simulink model "decibel"  (R2018a)
settings: Solver=VariableStepAuto  StartTime=0.0  StopTime=10e-3  RelTol=1e-3
libraries: simulink x1
settings Model: Creator=alex8  LastModifiedBy=alex8
settings OptimizationCC: DefaultParameterBehavior=Inlined  UseDivisionForNetSlopeComputation=on  UseFloatMulNetSlope=on  UseSpecifiedMinMax=on  InlineInvariantSignals=on  PassReuseOutputArgsAs=Individual arguments  ZeroExternalMemoryAtStartup=off  ZeroInternalMemoryAtStartup=off  NoFixptDivByZeroProtection=on  EfficientFloat2IntCast=on  LifeSpan=1  OptimizeBlockOrder=speed  DifferentSizesBufferReuse=on
settings DebuggingCC: ParameterTunabilityLossMsg=error
settings HardwareCC: ProdBitPerPointer=32  ProdBitPerSizeT=32  ProdBitPerPtrDiffT=32  ProdLargestAtomicInteger=Long  ProdLargestAtomicFloat=Double  ProdWordSize=32  ProdLongLongMode=on  ProdHWDeviceType=ARM Compatible->ARM Cortex
settings SFSimCC: MATLABDynamicMemAlloc=off
settings RTWCC: SystemTargetFile=ert.tlc  TemplateMakefile=ert_default_tmf  GenerateReport=on  BuildConfiguration=Faster Runs  IncludeHyperlinkInReport=on  LaunchReport=on  GenerateTraceInfo=on  GenerateTraceReport=on  GenerateTraceReportSl=on  GenerateTraceReportSf=on  GenerateTraceReportEml=on  GenerateCodeMetricsReport=on
settings CodeAppCC: ForceParamTrailComments=on  IgnoreCustomStorageClasses=off  OperatorAnnotations=on  SimulinkDataObjDesc=on  SFDataObjDesc=on  CustomSymbolStrGlobalVar=rt$N$M  CustomSymbolStrType=$N$M  CustomSymbolStrFcn=$N$M$F  CustomSymbolStrMacro=$N$M  InsertBlockDesc=on
settings ERTTargetCC: TargetLangStandard=C99 (ISO)  GenerateSampleERTMain=on  IncludeMdlTerminateFcn=off  CombineSignalStateStructs=on  SupportNonFinite=off  SupportComplex=off  SupportContinuousTime=on  InlinedParameterPlacement=NonHierarchical  ERTCustomFileTemplate=example_file_process.tlc  ERTFilePackagingFormat=CompactWithDataFile

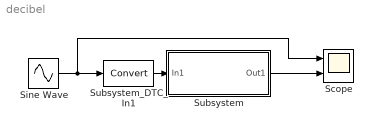
== system decibel ==
  Scope : Scope  NumInputPorts=2
  Sine Wave : Sin  Frequency=2*pi*1e3  SampleTime=0
  Subsystem : Subsystem
  Subsystem_DTC_In1 : DataTypeConversion
  wires:
  Sine Wave/1 -> Subsystem_DTC_In1/1, Scope/1
  Subsystem/1(Out1) -> Scope/2
  Subsystem_DTC_In1/1 -> Subsystem/1(In1)

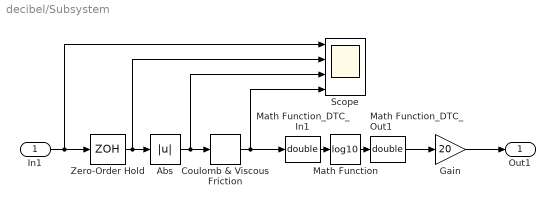
== system decibel/Subsystem ==
  In1 : Inport  OutDataTypeStr=fixdt(1,32,31)
  Abs : Abs  OutDataTypeStr=fixdt(0,32,31)
  Coulomb & Viscous Friction : simulink/Discontinuities/Coulomb & Viscous Friction  offset=1e-4  gain=1
      settings: SourceProductName=Simulink
  Gain : Gain  Gain=20
  Math Function : Math  Operator=log10  SaturateOnIntegerOverflow=on
  Math Function_DTC_In1 : DataTypeConversion  Tag=InsertedToIsolateUnsupportedBlock  OutDataTypeStr=double  LockScale=on
  Math Function_DTC_Out1 : DataTypeConversion  OutDataTypeStr=double
  Scope : Scope  NumInputPorts=4
  Zero-Order Hold : ZeroOrderHold  SampleTime=1/44100
  Out1 : Outport
  wires:
  In1/1 -> Scope/1, Zero-Order Hold/1
  Math Function/1 -> Math Function_DTC_Out1/1
  Gain/1 -> Out1/1
  Zero-Order Hold/1 -> Scope/2, Abs/1
  Abs/1 -> Scope/3, Coulomb & Viscous Friction/1
  Coulomb & Viscous Friction/1 -> Math Function_DTC_In1/1, Scope/4
  Math Function_DTC_In1/1 -> Math Function/1
  Math Function_DTC_Out1/1 -> Gain/1
